simulink model "Plant_2"  (R2024b)
settings: Solver=FixedStepAuto  StartTime=0.0  StopTime=10.0  FixedStep=0.02  RelTol=1e-3
values from neighbouring files (symbols this model uses):
  A = zeros(4, 4)    [Initialise_var_0.m]
  B = zeros(4, 2)    [Initialise_var_0.m]
  K = place(A, B, desired_poles)    [leunberger_obs_1.m]    (also in state_feedback.m; state_feedback_0.m; state_feedback_3.m; state_feedback_4.m = lqr(A,B,Q,R))
  L1 = 0.095    [Initialise_var_0.m]
  L2 = 0.095    [Initialise_var_0.m]
settings Model: Creator=Sez26  LastModifiedBy=Sez26

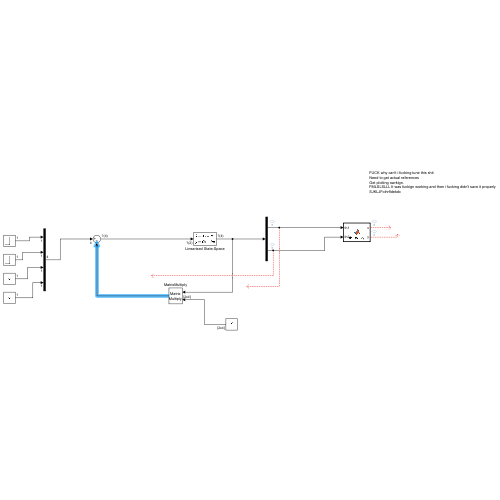
[thumbnail: Simulink's stored preview of the top-level diagram]
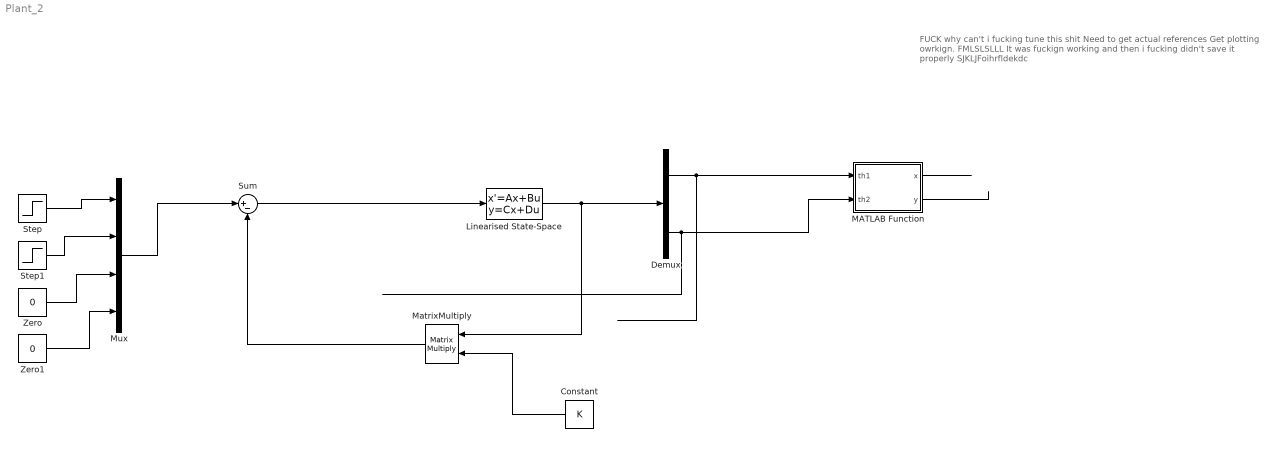
== system Plant_2 ==
  note: FUCK why can't i fucking tune this shit
      | Need to get actual references
      | Get plotting owrkign.
      | FMLSLSLLL It was fuckign working and then i fucking didn't save it properly
      | SJKLJFoihrfldekdc
  Constant : Constant  Value=K
  Demux : Demux  Outputs=2
  Linearised State-Space : StateSpace  A=A  B=B  C=[1 0 0 0; 0 1 0 0; 0 0 1 0; 0 0 0 1]  D=[0 0; 0 0; 0 0;0 0]  InitialCondition=0
  MATLAB Function : MATLAB Function  TreatAsAtomicUnit=on
  MatrixMultiply : Product  Multiplication=Matrix(*)
  Mux : Mux
  Step : Step  SampleTime=0
  Step1 : Step  SampleTime=0
  Sum : Sum  Inputs=|+-
  Zero : Constant  Value=0  OutDataTypeStr=Inherit: Inherit via back propagation
  Zero1 : Constant  Value=0  OutDataTypeStr=Inherit: Inherit via back propagation
  wires:
  Demux/1 -> MATLAB Function/1(th1)
  Demux/2 -> MATLAB Function/2(th2)
  MATLAB Function/1(x) -> ?
  MATLAB Function/2(y) -> ?
  Linearised State-Space/1 -> MatrixMultiply/1, Demux/1
  Constant/1 -> MatrixMultiply/2
  MatrixMultiply/1 -> Sum/2
  Step/1 -> Mux/1
  Step1/1 -> Mux/2
  Zero/1 -> Mux/3
  Zero1/1 -> Mux/4
  Mux/1 -> Sum/1
  Sum/1 -> Linearised State-Space/1

== matlab function Plant_2/MATLAB Function ==
  data: x output; th1 input; y output; th2 input; L1 parameter; L2 parameter
function [x,y] = th_to_xy(th1, th2, L1, L2)
    x = L1*cos(th1) + L2*cos(th2);
    y = L1*sin(th1) + L2*sin(th2);
